simulink model "sampleModel69"  (R2021b)
settings: Solver=VariableStepAuto  StartTime=0.0  StopTime=10.0  RelTol=1e-3
undefined symbols (not defined in the file or in its folder): DiscIntNeverNeededParam, Newton, Raphson
libraries: simulink x7
settings Model: Creator=user  LastModifiedBy=user

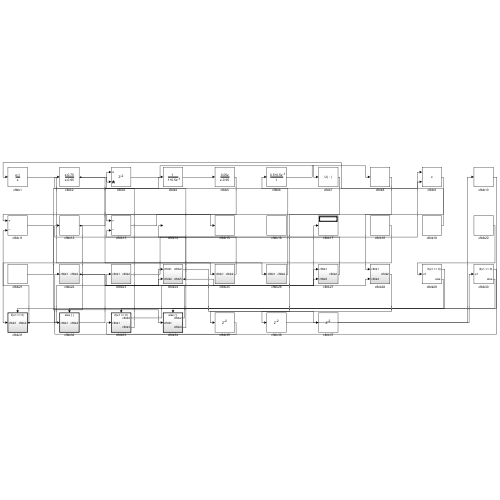
[thumbnail: Simulink's stored preview of the top-level diagram]
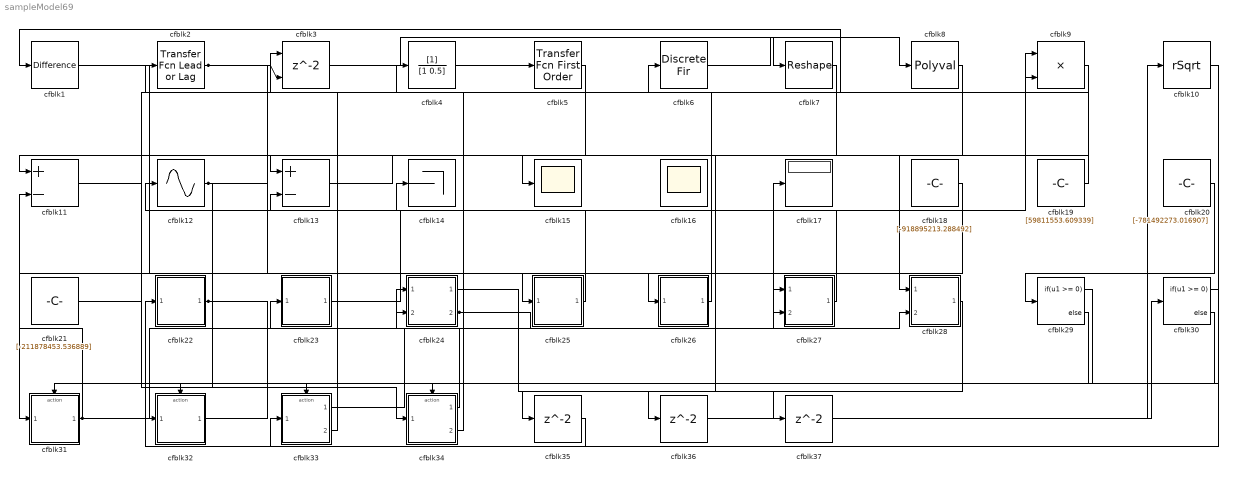
== system sampleModel69 ==
  cfblk1 : simulink/Discrete/Difference  ICPrevInput=0.0  OutMin=[]  OutMax=[]  OutDataTypeStr=Inherit: Inherit via back propagation  OutDataType=fixdt(1, 16)  OutScaling=2^-10  DoSatur=off
  cfblk10 : Sqrt  Operator=rSqrt  AlgorithmType=Newton-Raphson  SaturateOnIntegerOverflow=on
  cfblk11 : Sum  Inputs=+-
  cfblk12 : Sin  TimeSource=Use external signal  SampleTime=0
  cfblk13 : Sum  Inputs=+-
  cfblk14 : Terminator
  cfblk15 : Scope
  cfblk16 : Scope
      settings: Floating=on
  cfblk17 : Display
  cfblk18 : Constant  Value=[-918895213.288492]  SampleTime=1
  cfblk19 : Constant  Value=[59811553.609339]  SampleTime=1
  cfblk2 : simulink/Discrete/Transfer Fcn Lead or Lag  PoleZ=0.95  ZeroZ=0.75  ICPrevOutput=0.0  ICPrevInput=0.0  DoSatur=off
      settings: SourceProductBaseCode=SL
  cfblk20 : Constant  Value=[-781492273.016907]  SampleTime=1
  cfblk21 : Constant  Value=[-211878453.536889]  SampleTime=1
  cfblk22 : Subsystem
  cfblk23 : Subsystem
  cfblk24 : Subsystem
  cfblk25 : Subsystem
  cfblk26 : Subsystem
  cfblk27 : Subsystem
  cfblk28 : Subsystem
  cfblk29 : If  IfExpression=u1 >= 0  SampleTime=1
  cfblk3 : Delay  ShowEnablePort=on  SampleTime=1
      settings: InputPortMap=u0,e6
  cfblk30 : If  IfExpression=u1 >= 0  SampleTime=1
  cfblk31 : Subsystem  TreatAsAtomicUnit=on
  cfblk32 : Subsystem  TreatAsAtomicUnit=on
  cfblk33 : Subsystem  TreatAsAtomicUnit=on
  cfblk34 : Subsystem  TreatAsAtomicUnit=on
  cfblk35 : Delay  SampleTime=1
  cfblk36 : Delay  SampleTime=1
  cfblk37 : Delay  SampleTime=1
  cfblk4 : DiscreteFilter  SampleTime=1
  cfblk5 : simulink/Discrete/Transfer Fcn First Order  PoleZ=0.95  ICPrevOutput=0.0  DoSatur=off
  cfblk6 : DiscreteFir  SampleTime=1
  cfblk7 : Reshape
  cfblk8 : Polyval  Coefs=[ +2.081618890e-019, -1.441693666e-014, +4.719686976e-010, -8.536869453e-006, +1.621573104e-001, -8.087801117e+001 ]
  cfblk9 : Product  Inputs=**
  wires:
  cfblk34/1(cfblk2) -> cfblk23/1(cfblk1)
  cfblk27/1(cfblk2) -> cfblk14/1
  cfblk1/1 -> cfblk25/1(cfblk1)
  cfblk34/2(cfblk4) -> cfblk3/1
  cfblk3/1 -> cfblk7/1
  cfblk19/1 -> cfblk1/1
  cfblk26/1(cfblk2) -> cfblk6/1
  cfblk10/1 -> cfblk22/1(cfblk1)
  cfblk13/1 -> cfblk15/1
  cfblk33/1(cfblk2) -> cfblk17/1
  cfblk2/1 -> cfblk3/2, cfblk26/1(cfblk1)
  cfblk23/1(cfblk2) -> cfblk9/1
  cfblk25/1(cfblk2) -> cfblk12/1
  cfblk5/1 -> cfblk11/1
  cfblk31/1(cfblk2) -> cfblk11/2, cfblk24/1(cfblk1)
  cfblk20/1 -> cfblk29/1
  cfblk21/1 -> cfblk9/2
  cfblk7/1 -> cfblk13/1
  cfblk33/2(cfblk3) -> cfblk2/1
  cfblk18/1 -> cfblk31/1(cfblk1)
  cfblk6/1 -> cfblk8/1
  cfblk12/1 -> cfblk4/1, cfblk32/1(cfblk1)
  cfblk8/1 -> cfblk28/1(cfblk1)
  cfblk4/1 -> cfblk5/1
  cfblk22/1(cfblk2) -> cfblk28/2(cfblk4), cfblk24/2(cfblk4)
  cfblk24/2(cfblk5) -> cfblk27/1(cfblk1), cfblk13/2
  cfblk32/1(cfblk2) -> cfblk27/2(cfblk5)
  cfblk11/1 -> cfblk34/1(cfblk1)
  cfblk29/1 -> cfblk31/Action
  cfblk29/2 -> cfblk32/Action
  cfblk30/1 -> cfblk33/Action
  cfblk30/2 -> cfblk34/Action
  cfblk28/1(cfblk2) -> cfblk35/1
  cfblk35/1 -> cfblk33/1(cfblk1)
  cfblk9/1 -> cfblk36/1
  cfblk36/1 -> cfblk30/1
  cfblk24/1(cfblk2) -> cfblk37/1
  cfblk37/1 -> cfblk10/1

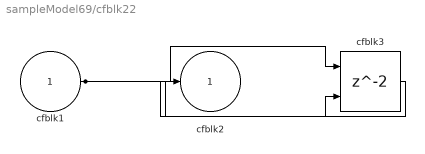
== system sampleModel69/cfblk22 ==
  cfblk1 : Inport
  cfblk3 : Delay  ShowEnablePort=on  SampleTime=1
      settings: InputPortMap=u0,e6
  cfblk2 : Outport
  wires:
  cfblk1/1 -> cfblk3/1, cfblk3/2
  cfblk3/1 -> cfblk2/1

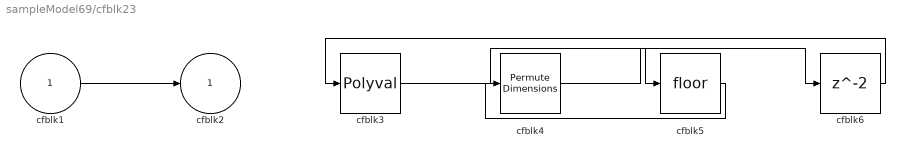
== system sampleModel69/cfblk23 ==
  cfblk1 : Inport
  cfblk3 : Polyval  Coefs=[ +2.081618890e-019, -1.441693666e-014, +4.719686976e-010, -8.536869453e-006, +1.621573104e-001, -8.087801117e+001 ]
  cfblk4 : PermuteDimensions
  cfblk5 : Rounding
  cfblk6 : Delay  SampleTime=1
  cfblk2 : Outport
  wires:
  cfblk1/1 -> cfblk2/1
  cfblk3/1 -> cfblk5/1
  cfblk5/1 -> cfblk4/1
  cfblk4/1 -> cfblk6/1
  cfblk6/1 -> cfblk3/1

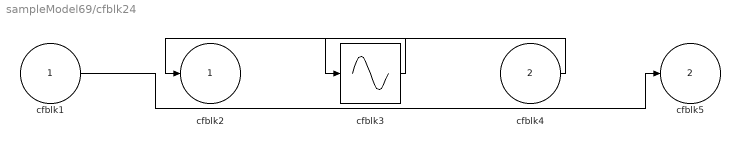
== system sampleModel69/cfblk24 ==
  cfblk1 : Inport
  cfblk4 : Inport  Port=2
  cfblk3 : Sin  TimeSource=Use external signal  SampleTime=0
  cfblk2 : Outport
  cfblk5 : Outport  Port=2
  wires:
  cfblk3/1 -> cfblk2/1
  cfblk1/1 -> cfblk5/1
  cfblk4/1 -> cfblk3/1

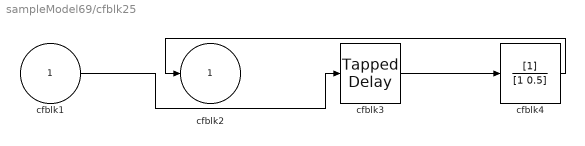
== system sampleModel69/cfblk25 ==
  cfblk1 : Inport
  cfblk3 : simulink/Discrete/Tapped Delay  vinit=0.0  samptime=-1  NumDelays=1  DelayOrder=Oldest  includeCurrent=off
  cfblk4 : DiscreteFilter  SampleTime=1
  cfblk2 : Outport
  wires:
  cfblk3/1 -> cfblk4/1
  cfblk4/1 -> cfblk2/1
  cfblk1/1 -> cfblk3/1

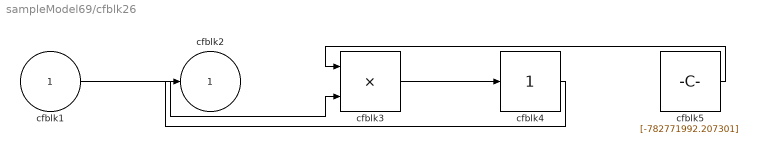
== system sampleModel69/cfblk26 ==
  cfblk1 : Inport
  cfblk3 : Product
  cfblk4 : simulink/Math Operations/Slider Gain  gain=1  low=0  high=2
  cfblk5 : Constant  Value=[-782771992.207301]  SampleTime=1
  cfblk2 : Outport
  wires:
  cfblk5/1 -> cfblk3/1
  cfblk1/1 -> cfblk3/2
  cfblk3/1 -> cfblk4/1
  cfblk4/1 -> cfblk2/1

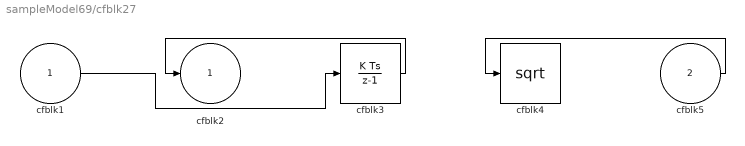
== system sampleModel69/cfblk27 ==
  cfblk1 : Inport
  cfblk5 : Inport  Port=2
  cfblk3 : DiscreteIntegrator  ICPrevOutput=DiscIntNeverNeededParam  ICPrevScaledInput=DiscIntNeverNeededParam
  cfblk4 : Sqrt  SaturateOnIntegerOverflow=on
  cfblk2 : Outport
  wires:
  cfblk3/1 -> cfblk2/1
  cfblk1/1 -> cfblk3/1
  cfblk5/1 -> cfblk4/1

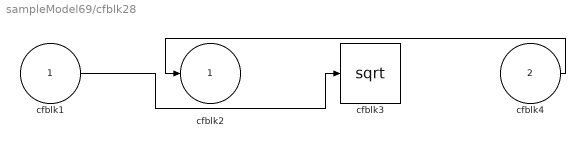
== system sampleModel69/cfblk28 ==
  cfblk1 : Inport
  cfblk4 : Inport  Port=2
  cfblk3 : Sqrt  SaturateOnIntegerOverflow=on
  cfblk2 : Outport
  wires:
  cfblk4/1 -> cfblk2/1
  cfblk1/1 -> cfblk3/1

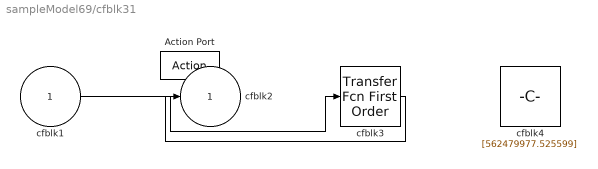
== system sampleModel69/cfblk31 ==
  cfblk1 : Inport
  Action Port : ActionPort  ActionPortLabel=if(u1 >= 0)
  cfblk3 : simulink/Discrete/Transfer Fcn First Order  PoleZ=0.95  ICPrevOutput=0.0  DoSatur=off
  cfblk4 : Constant  Value=[562479977.525599]  SampleTime=1
  cfblk2 : Outport
  wires:
  cfblk1/1 -> cfblk3/1
  cfblk3/1 -> cfblk2/1

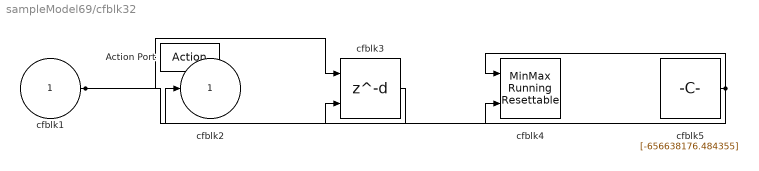
== system sampleModel69/cfblk32 ==
  cfblk1 : Inport
  Action Port : ActionPort  ActionPortLabel=else
  cfblk3 : Delay  DelayLengthSource=Input port
      settings: InputPortMap=u0,p1
  cfblk4 : simulink/Math Operations/MinMax Running Resettable  Function=min  vinit=0.0
  cfblk5 : Constant  Value=[-656638176.484355]  SampleTime=1
  cfblk2 : Outport
  wires:
  cfblk3/1 -> cfblk2/1
  cfblk1/1 -> cfblk3/1, cfblk4/2
  cfblk5/1 -> cfblk3/2, cfblk4/1

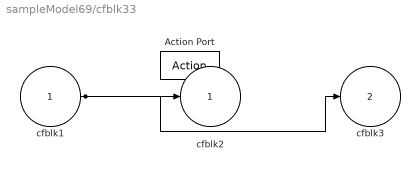
== system sampleModel69/cfblk33 ==
  cfblk1 : Inport
  Action Port : ActionPort  ActionPortLabel=if(u1 >= 0)
  cfblk2 : Outport
  cfblk3 : Outport  Port=2
  wires:
  cfblk1/1 -> cfblk2/1, cfblk3/1

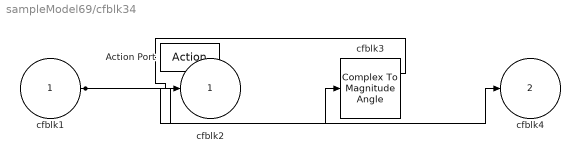
== system sampleModel69/cfblk34 ==
  cfblk1 : Inport
  Action Port : ActionPort  ActionPortLabel=else
  cfblk3 : ComplexToMagnitudeAngle
  cfblk2 : Outport
  cfblk4 : Outport  Port=2
  wires:
  cfblk1/1 -> cfblk4/1, cfblk3/1
  cfblk3/1 -> cfblk2/1
